simulink model "Demo1_P1A3"  (R2023a)
settings: Solver=VariableStepAuto  StartTime=0.0  StopTime=10.0  RelTol=1e-3
settings Model: Creator=rqouta  LastModifiedBy=rqouta

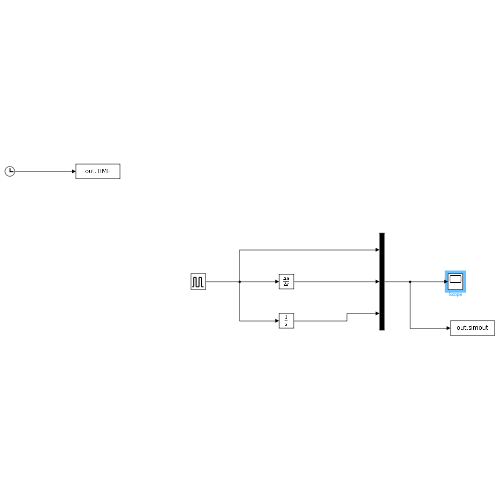
[thumbnail: Simulink's stored preview of the top-level diagram]
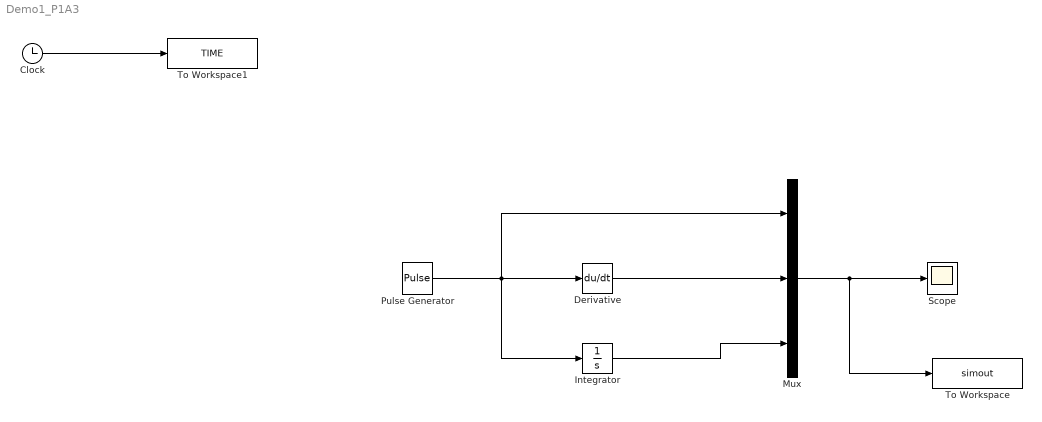
== system Demo1_P1A3 ==
  Clock : Clock
  Derivative : Derivative
  Integrator : Integrator
  Mux : Mux  Inputs=3
  Pulse Generator : DiscretePulseGenerator  PulseType=Time based  Period=5  PulseWidth=50
  Scope : Scope
  To Workspace : ToWorkspace  VariableName=simout  SampleTime=-1
  To Workspace1 : ToWorkspace  VariableName=TIME  SampleTime=-1
  wires:
  Integrator/1 -> Mux/3
  Mux/1 -> To Workspace/1, Scope/1
  Pulse Generator/1 -> Mux/1, Integrator/1, Derivative/1
  Derivative/1 -> Mux/2
  Clock/1 -> To Workspace1/1
